simulink model "Model_3"  (Simulink 9.2)
settings: Solver=VariableStepAuto  StartTime=0.0  StopTime=10.0  RelTol=1e-3
settings Model: Creator=Dravius  LastModifiedBy=Dravius
settings DataIOCC: LimitDataPoints=off  SaveFormat=Dataset  SignalLoggingSaveFormat=Dataset
settings OptimizationCC: LifeSpan=auto
settings DebuggingCC: UnderspecifiedInitializationDetection=Simplified  MergeDetectMultiDrivingBlocksExec=error  FcnCallInpInsideContextMsg=error  StateNameClashWarn=none  SFUnexpectedBacktrackingDiag=error  SFNoUnconditionalDefaultTransitionDiag=error  SFExecutionAtInitializationDiag=warning
settings HardwareCC: ProdBitPerPointer=64  ProdBitPerSizeT=64  ProdBitPerPtrDiffT=64  ProdLargestAtomicFloat=Float  ProdIntDivRoundTo=Zero  ProdEndianess=LittleEndian  ProdWordSize=64  ProdHWDeviceType=Intel->x86-64 (Windows64)
settings ModelReferenceCC: PropagateSignalLabelsOutOfModel=on
settings SFSimCC: SimUseLocalCustomCode=on
settings RTWCC: RTWUseLocalCustomCode=on
settings CodeAppCC: StateflowObjectComments=off
settings GRTTargetCC: TargetLangStandard=C99 (ISO)  GeneratePreprocessorConditionals=Use local settings  CombineOutputUpdateFcns=on  GRTInterface=off
settings ConfigComp: CovMetricSettings=dwe  CovHtmlReporting=off  CovSaveCumulativeToWorkspaceVar=off  CovSaveSingleToWorkspaceVar=off  CovExternalEMLEnable=on

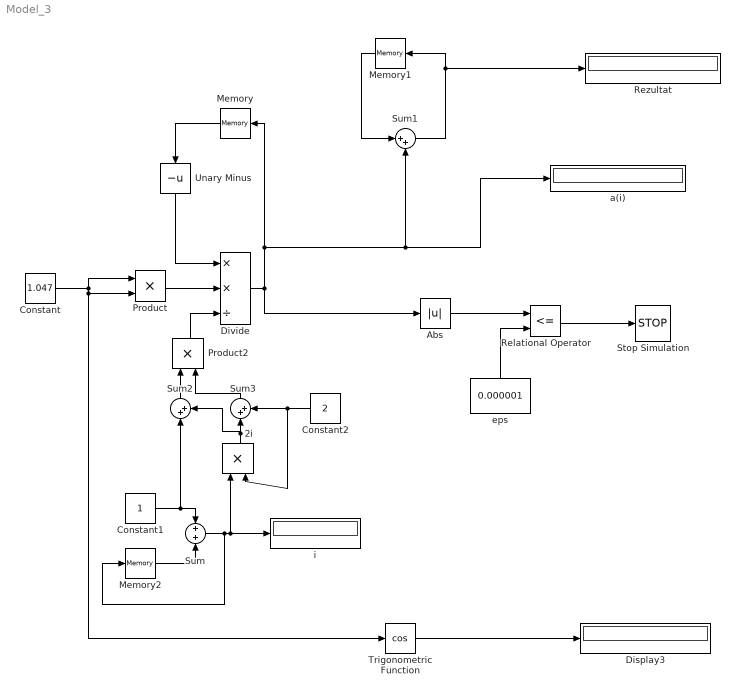
== system Model_3 ==
  2i : Product
  Abs : Abs
  Constant : Constant  Value=1.047
  Constant1 : Constant
  Constant2 : Constant  Value=2
  Display3 : Display
  Divide : Product  Inputs=**/
  Memory : Memory  InitialCondition=1
  Memory1 : Memory  InitialCondition=1
  Memory2 : Memory  InitialCondition=-1
  Product : Product
  Product2 : Product
  Relational Operator : RelationalOperator  Operator=<=  OutDataTypeStr=boolean  RndMeth=Simplest
  Rezultat : Display
  Stop Simulation : Stop
  Sum : Sum
  Sum1 : Sum  Inputs=|++
  Sum2 : Sum  Inputs=|++
  Sum3 : Sum  Inputs=|++
  Trigonometric Function : Trigonometry  Operator=cos
  Unary Minus : UnaryMinus
  a(i) : Display
  eps : Constant  Value=0.000001
  i : Display
  wires:
  Constant/1 -> Product/2, Trigonometric Function/1, Product/1
  Constant1/1 -> Sum2/1, Sum/1
  Memory2/1 -> Sum/2
  Sum/1 -> 2i/1, i/1, Memory2/1
  Memory/1 -> Unary Minus/1
  Divide/1 -> a(i)/1, Sum1/2, Memory/1, Abs/1
  Sum1/1 -> Rezultat/1, Memory1/1
  Memory1/1 -> Sum1/1
  Abs/1 -> Relational Operator/1
  Relational Operator/1 -> Stop Simulation/1
  eps/1 -> Relational Operator/2
  Trigonometric Function/1 -> Display3/1
  Product/1 -> Divide/2
  Unary Minus/1 -> Divide/1
  Product2/1 -> Divide/3
  Constant2/1 -> 2i/2, Sum3/2
  2i/1 -> Sum2/2, Sum3/1
  Sum3/1 -> Product2/2
  Sum2/1 -> Product2/1
